simulink model "smlkT1"  (R2022a)
settings: Solver=VariableStepAuto  StartTime=0.0  StopTime=10.0  MaxStep=0.0001  RelTol=1e-3
values from neighbouring files (symbols this model uses):
  g = 9.81    [Tarea1_SeminarioDeModelado.m]
  L1 = 0.3    [Tarea1_SeminarioDeModelado.m]
  L2 = 0.25    [Tarea1_SeminarioDeModelado.m]
  m1 = 0.2    [Tarea1_SeminarioDeModelado.m]
  m2 = 0.1    [Tarea1_SeminarioDeModelado.m]
settings Model: Creator=julio  LastModifiedBy=julio

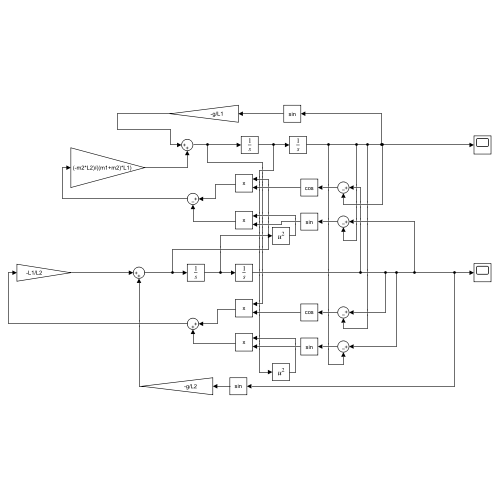
[thumbnail: Simulink's stored preview of the top-level diagram]
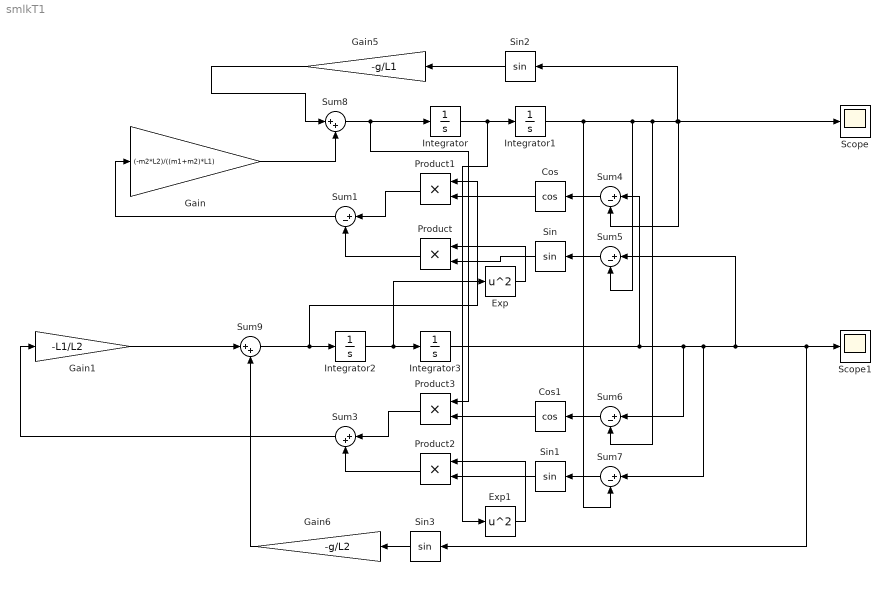
== system smlkT1 ==
  Cos : Trigonometry  Operator=cos
  Cos1 : Trigonometry  Operator=cos
  Exp : Math  Operator=square
  Exp1 : Math  Operator=square
  Gain : Gain  Gain=(-m2*L2)/((m1+m2)*L1)
  Gain1 : Gain  Gain=-L1/L2
  Gain5 : Gain  Gain=-g/L1
  Gain6 : Gain  Gain=-g/L2
  Integrator : Integrator
  Integrator1 : Integrator
  Integrator2 : Integrator
  Integrator3 : Integrator  InitialCondition=0.61
  Product{,1..3} (4 alike) : Product
  Scope : Scope
  Scope1 : Scope
  Sin{,1..3} (4 alike) : Trigonometry
  Sum{1,4..7} (5 alike) : Sum  Inputs=|+-
  Sum3 : Sum  Inputs=|++
  Sum8 : Sum  Inputs=|++
  Sum9 : Sum  Inputs=|++
  wires:
  Integrator/1 -> Exp1/1, Integrator1/1
  Integrator1/1 -> Sum7/2, Sin2/1, Scope/1, Sum4/2, Sum6/2, Sum5/2
  Product/1 -> Sum1/2
  Product1/1 -> Sum1/1
  Sin/1 -> Product/2
  Cos/1 -> Product1/2
  Sum1/1 -> Gain/1
  Sum3/1 -> Gain1/1
  Product2/1 -> Sum3/2
  Cos1/1 -> Product3/2
  Sin1/1 -> Product2/2
  Integrator3/1 -> Sum4/1, Sum6/1, Sum7/1, Sum5/1, Sin3/1, Scope1/1
  Integrator2/1 -> Exp/1, Integrator3/1
  Exp/1 -> Product/1
  Sum4/1 -> Cos/1
  Sum5/1 -> Sin/1
  Sum7/1 -> Sin1/1
  Sum6/1 -> Cos1/1
  Exp1/1 -> Product2/1
  Sin2/1 -> Gain5/1
  Sin3/1 -> Gain6/1
  Product3/1 -> Sum3/1
  Gain5/1 -> Sum8/1
  Sum8/1 -> Product3/1, Integrator/1
  Gain1/1 -> Sum9/1
  Sum9/1 -> Product1/1, Integrator2/1
  Gain6/1 -> Sum9/2
  Gain/1 -> Sum8/2
